simulink model "crazyflie_241010"  (R2024b)
settings: Solver=VariableStepAuto  StartTime=0.0  StopTime=10.0  RelTol=1e-3
model workspace (MAT data in the model file):
  CONFIG_CONTROLLER_PID_FILTER_ALL = Simulink.Parameter
  CONFIG_CONTROLLER_PID_FILTER_ALL.Complexity = 'real'
  CONFIG_CONTROLLER_PID_FILTER_ALL.Dimensions = [0 0]
  CONFIG_CONTROLLER_PID_FILTER_ALL.DataType = 'auto'
  a1 = Simulink.Parameter
  a1.Value = 2
  a1.Complexity = 'real'
  a1.Dimensions = [1 1]
  a1.DataType = 'auto'
  a2 = Simulink.Parameter
  a2.Value = 3
  a2.Complexity = 'real'
  a2.Dimensions = [1 1]
  a2.DataType = 'auto'
  b0 = Simulink.Parameter
  b0.Value = 5
  b0.Complexity = 'real'
  b0.Dimensions = [1 1]
  b0.DataType = 'auto'
  b1 = Simulink.Parameter
  b1.Value = 7
  b1.Complexity = 'real'
  b1.Dimensions = [1 1]
  b1.DataType = 'auto'
  b2 = Simulink.Parameter
  b2.Value = 11
  b2.Complexity = 'real'
  b2.Dimensions = [1 1]
  b2.DataType = 'auto'
  pid_dt = Simulink.Parameter
  pid_dt.Complexity = 'real'
  pid_dt.Dimensions = [0 0]
  pid_dt.DataType = 'auto'
  pid_enableDFilter = Simulink.Parameter
  pid_enableDFilter.Complexity = 'real'
  pid_enableDFilter.Dimensions = [0 0]
  pid_enableDFilter.DataType = 'auto'
  pid_iLimit = Simulink.Parameter
  pid_iLimit.Complexity = 'real'
  pid_iLimit.Dimensions = [0 0]
  pid_iLimit.DataType = 'auto'
  pid_kd = Simulink.Parameter
  pid_kd.Complexity = 'real'
  pid_kd.Dimensions = [0 0]
  pid_kd.DataType = 'auto'
  pid_kff = Simulink.Parameter
  pid_kff.Complexity = 'real'
  pid_kff.Dimensions = [0 0]
  pid_kff.DataType = 'auto'
  pid_ki = Simulink.Parameter
  pid_ki.Complexity = 'real'
  pid_ki.Dimensions = [0 0]
  pid_ki.DataType = 'auto'
  pid_kp = Simulink.Parameter
  pid_kp.Complexity = 'real'
  pid_kp.Dimensions = [0 0]
  pid_kp.DataType = 'auto'
  pid_outputLimit = Simulink.Parameter
  pid_outputLimit.Complexity = 'real'
  pid_outputLimit.Dimensions = [0 0]
  pid_outputLimit.DataType = 'auto'
settings Model: Creator=thomas  LastModifiedBy=thomas

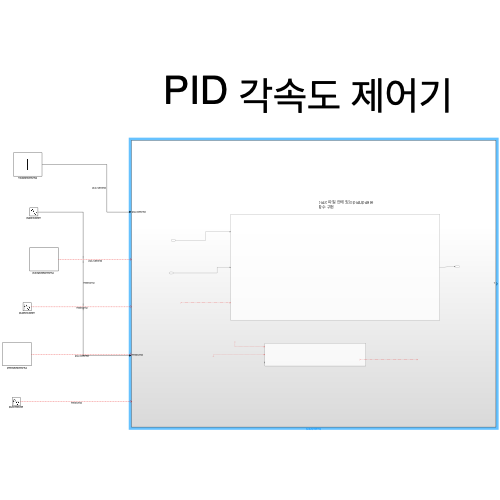
[thumbnail: Simulink's stored preview of the top-level diagram]
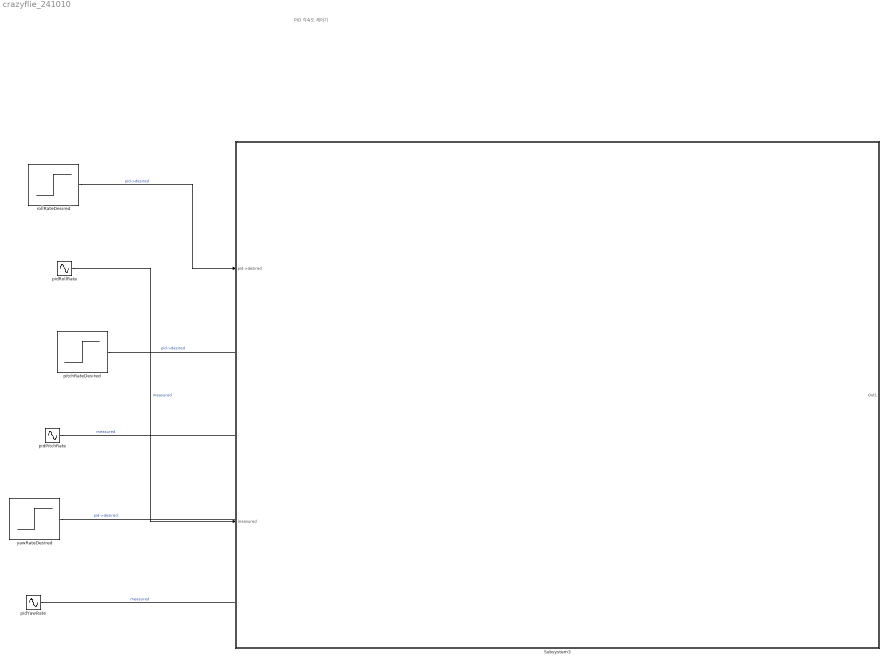
== system crazyflie_241010 ==
  note: PID 각속도 제어기
  Subsystem3 : Subsystem
  pidPitchRate : Sin  SampleTime=0
  pidRollRate : Sin  SampleTime=0
  pidYawRate : Sin  SampleTime=0
  "pitchRateDesired  " : Step  SampleTime=0
  rollRateDesired : Step  SampleTime=0
  yawRateDesired : Step  SampleTime=0
  wires:
  rollRateDesired/1 -> Subsystem3/1(pid->desired)  "pid->desired"
  pidRollRate/1 -> Subsystem3/2(measured)  "measured"
  "pitchRateDesired  "/1 -> ?  "pid->desired"
  pidPitchRate/1 -> ?  "measured"
  yawRateDesired/1 -> ?  "pid->desired"
  pidYawRate/1 -> ?  "measured"

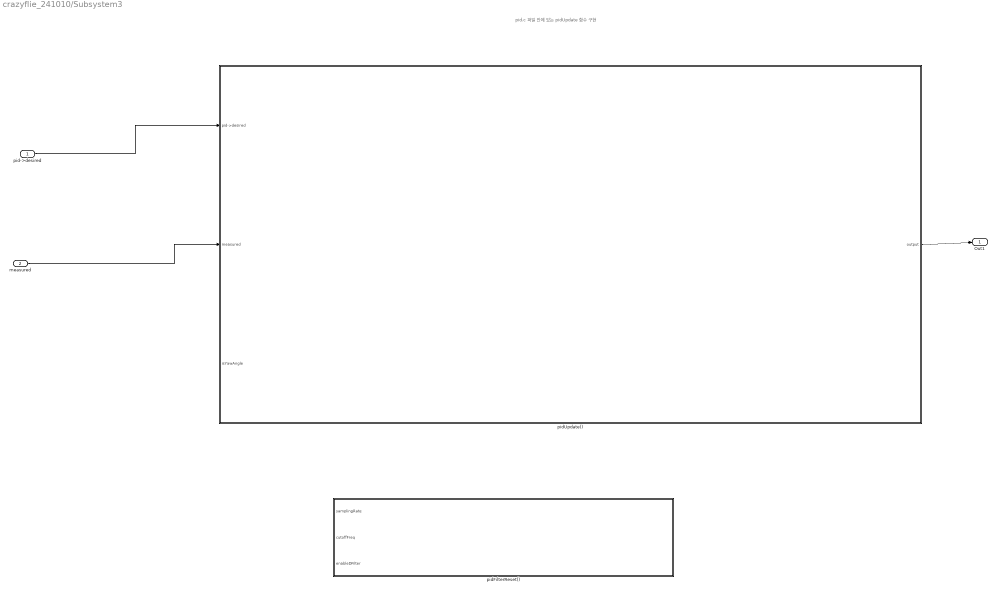
== system crazyflie_241010/Subsystem3 ==
  note: pid.c 파일 안에 있는 pidUpdate 함수 구현
  pid->desired : Inport
  measured : Inport  Port=2
  pidFilterReset() : Subsystem
  pidUpdate() : Subsystem
  Out1 : Outport
  wires:
  measured/1 -> pidUpdate()/2(measured)
  pid->desired/1 -> pidUpdate()/1(pid->desired)
  pidUpdate()/1(output) -> Out1/1
  ? -> pidUpdate()/3(isYawAngle)
  ? -> pidFilterReset()/1(samplingRate)
  ? -> ?
  ? -> pidFilterReset()/2(cutoffFreq)

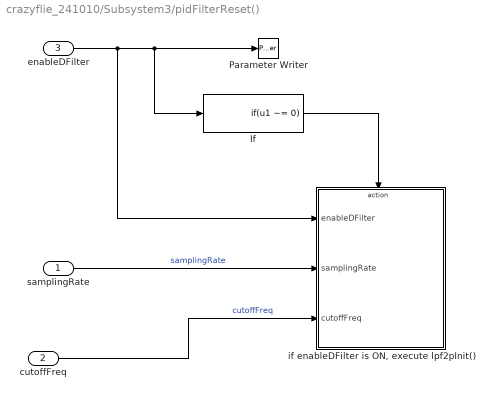
== system crazyflie_241010/Subsystem3/pidFilterReset() ==
  samplingRate : Inport
  cutoffFreq : Inport  Port=2
  enableDFilter : Inport  Port=3
  If : If  IfExpression=u1 ~= 0  ShowElse=off
  Parameter Writer : ParameterWriter  WorkspaceVariableName=pid_enableDFilter  Destination=Model workspace variable
  "if enableDFilter is ON, execute lpf2pInit()" : Subsystem  TreatAsAtomicUnit=on
  wires:
  samplingRate/1 -> "if enableDFilter is ON, execute lpf2pInit()"/2(samplingRate)  "samplingRate"
  enableDFilter/1 -> "if enableDFilter is ON, execute lpf2pInit()"/1(enableDFilter), If/1, Parameter Writer/1
  cutoffFreq/1 -> "if enableDFilter is ON, execute lpf2pInit()"/3(cutoffFreq)  "cutoffFreq"
  If/1 -> "if enableDFilter is ON, execute lpf2pInit()"/Action

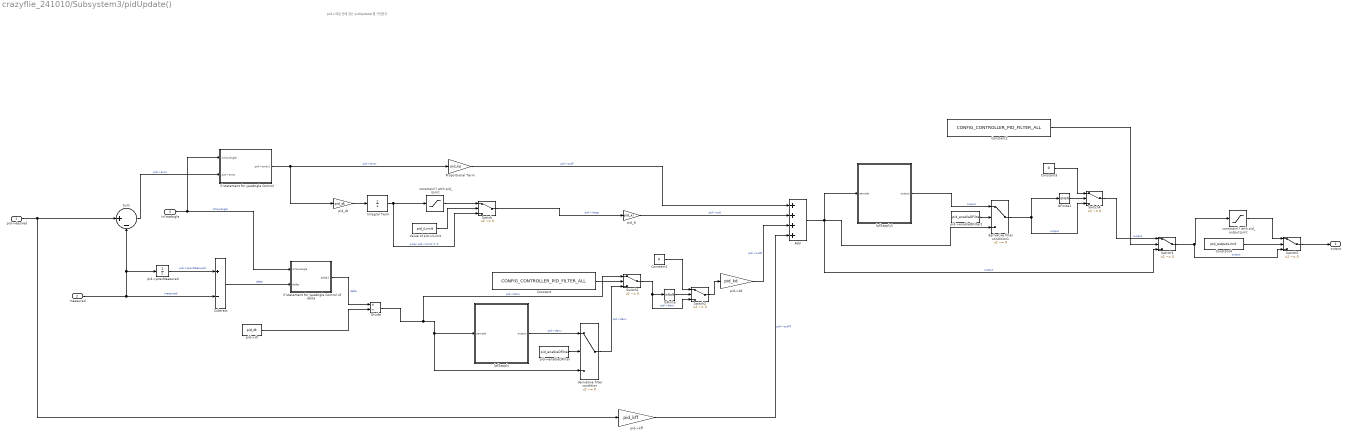
== system crazyflie_241010/Subsystem3/pidUpdate() ==
  note: pid.c 파일 안에 있는 pidUpdate()를 구현한것 .
  pid->desired : Inport
  measured : Inport  Port=2
  isYawAngle : Inport  Port=3
  Add : Sum  Inputs=++++
  Constant : Constant  Value=CONFIG_CONTROLLER_PID_FILTER_ALL
  Constant1 : Constant  Value=0
  Constant2 : Constant  Value=CONFIG_CONTROLLER_PID_FILTER_ALL
  Constant3 : Constant  Value=0
  Constant4 : Constant  Value=pid_outputLimit
  Divide : Product  Inputs=*/
  Integral Term : Integrator
  IsFinite : RelationalOperator  Operator=isNaN  OutDataTypeStr=boolean  RndMeth=Simplest  InputSameDT=off
  IsFinite1 : RelationalOperator  Operator=isNaN  OutDataTypeStr=boolean  RndMeth=Simplest  InputSameDT=off
  Proportional Term : Gain  Gain=pid_kp
  Subtract : Sum  Inputs=+-
  Sum : Sum  Inputs=|+-
  Switch{,1..5} (6 alike) : Switch  Criteria=u2 ~= 0  SaturateOnIntegerOverflow=off  InputSameDT=off
  Value of pid->iLimit : Constant  Value=pid_iLimit
  constrain() with pid_iLimit : Saturate  UpperLimit=pid_iLimit  LowerLimit=-pid_iLimit
  constrain() with pid_outputLimit : Saturate  UpperLimit=pid_outputLimit  LowerLimit=-pid_outputLimit
  derivative filter condition : Switch  Criteria=u2 ~= 0  Threshold=0.5  SaturateOnIntegerOverflow=off  InputSameDT=off
  derivative filter condition1 : Switch  Criteria=u2 ~= 0  Threshold=0.5  SaturateOnIntegerOverflow=off  InputSameDT=off
  "if statement for yawAngle Control " : Subsystem
  if statement for yawAngle Control of delta : Subsystem
  lpf2apply : Subsystem
  lpf2apply1 : Subsystem
  pid->dt : Constant  Value=pid_dt
  pid->enableDFilter : Constant  Value=pid_enableDFilter  LockScale=on
  pid->enableDFilter1 : Constant  Value=pid_enableDFilter  LockScale=on
  pid->kd : Gain  Gain=pid_kd
  pid->kff : Gain  Gain=pid_kff
  pid->prevMeasured : UnitDelay  SampleTime=-1  HasFrameUpgradeWarning=on
  pid_dt : Gain  Gain=pid_dt
  pid_ki : Gain  Gain=pid_ki
  output : Outport
  wires:
  pid->desired/1 -> pid->kff/1, Sum/1
  constrain() with pid_iLimit/1 -> Switch/1
  Integral Term/1 -> constrain() with pid_iLimit/1, Switch/3  "when pid->iLimit = 0"
  pid_dt/1 -> Integral Term/1
  pid->dt/1 -> Divide/2
  pid->kd/1 -> Add/3  "pid->outD"
  derivative filter condition/1 -> Switch1/3  "pid->deriv"
  Proportional Term/1 -> Add/1  "pid->outP"
  pid->prevMeasured/1 -> Subtract/1  "pid->prevMeasured"
  Value of pid->iLimit/1 -> Switch/2
  lpf2apply/1(output) -> derivative filter condition/1  "pid->deriv"
  Switch/1 -> pid_ki/1  "pid->integ"
  Subtract/1 -> if statement for yawAngle Control of delta/2(delta)  "delta"
  measured/1 -> Sum/2, pid->prevMeasured/1, Subtract/2  "measured"
  pid_ki/1 -> Add/2  "pid->outI"
  pid->enableDFilter/1 -> derivative filter condition/2
  "if statement for yawAngle Control "/1(pid->error1) -> Proportional Term/1, pid_dt/1  "pid->error"
  isYawAngle/1 -> "if statement for yawAngle Control "/1(isYawAngle), if statement for yawAngle Control of delta/1(isYawAngle)  "isYawAngle"
  Sum/1 -> "if statement for yawAngle Control "/2(pid->error)  "pid->error"
  if statement for yawAngle Control of delta/1(delta1) -> Divide/1  "delta"
  pid->kff/1 -> Add/4  "pid->outFF"
  Constant/1 -> Switch1/2
  Divide/1 -> derivative filter condition/3, lpf2apply/1(sample), Switch1/1  "pid->deriv"
  Switch1/1 -> Switch2/3, IsFinite/1  "pid->deriv"
  IsFinite/1 -> Switch2/2
  Constant1/1 -> Switch2/1
  Switch2/1 -> pid->kd/1
  Add/1 -> lpf2apply1/1(sample), derivative filter condition1/3, Switch3/3  "output"
  pid->enableDFilter1/1 -> derivative filter condition1/2
  Constant3/1 -> Switch4/1
  IsFinite1/1 -> Switch4/2
  lpf2apply1/1(output) -> derivative filter condition1/1  "output"
  derivative filter condition1/1 -> Switch4/3, IsFinite1/1  "output"
  Constant2/1 -> Switch3/2
  Switch4/1 -> Switch3/1  "output"
  Constant4/1 -> Switch5/2
  Switch3/1 -> Switch5/3, constrain() with pid_outputLimit/1  "output"
  constrain() with pid_outputLimit/1 -> Switch5/1
  Switch5/1 -> output/1

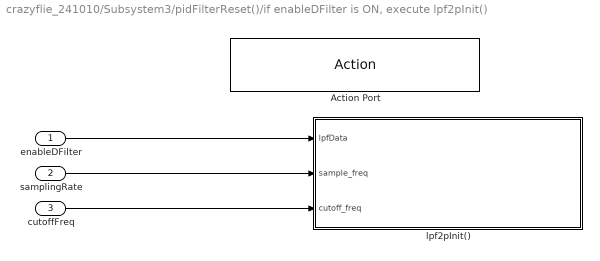
== system crazyflie_241010/Subsystem3/pidFilterReset()/if enableDFilter is ON, execute lpf2pInit() ==
  enableDFilter : Inport
  samplingRate : Inport  Port=2
  cutoffFreq : Inport  Port=3
  Action Port : ActionPort  ActionPortLabel=if(u1 ~= 0)
  lpf2pInit() : Subsystem
  wires:
  enableDFilter/1 -> lpf2pInit()/1(lpfData)
  samplingRate/1 -> lpf2pInit()/2(sample_freq)
  cutoffFreq/1 -> lpf2pInit()/3(cutoff_freq)

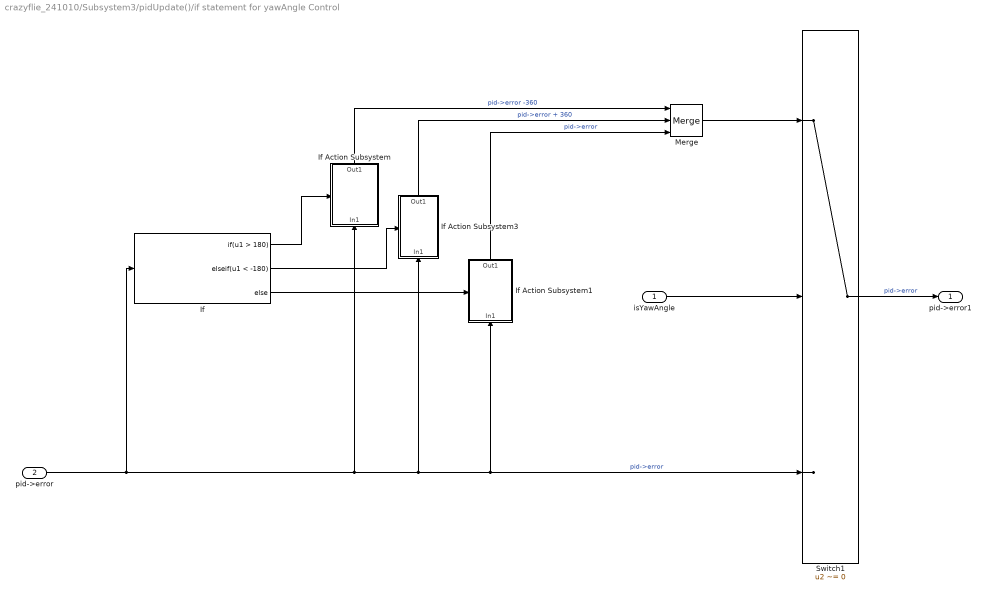
== system crazyflie_241010/Subsystem3/pidUpdate()/if statement for yawAngle Control  ==
  isYawAngle : Inport
  pid->error : Inport  Port=2
  If : If  IfExpression=u1 > 180  ElseIfExpressions=u1 < -180
  If Action Subsystem : Subsystem  TreatAsAtomicUnit=on
  If Action Subsystem1 : Subsystem  TreatAsAtomicUnit=on
  If Action Subsystem3 : Subsystem  TreatAsAtomicUnit=on
  Merge : Merge  Inputs=3
  Switch1 : Switch  Criteria=u2 ~= 0  Threshold=0.5  SaturateOnIntegerOverflow=off  InputSameDT=off
  pid->error1 : Outport
  wires:
  If Action Subsystem3/1(Out1) -> Merge/2  "pid->error + 360"
  Merge/1 -> Switch1/1
  Switch1/1 -> pid->error1/1  "pid->error"
  isYawAngle/1 -> Switch1/2
  pid->error/1 -> If Action Subsystem1/1(In1), Switch1/3, If Action Subsystem3/1(In1), If Action Subsystem/1(In1), If/1  "pid->error"
  If/3 -> If Action Subsystem1/Action
  If Action Subsystem1/1(Out1) -> Merge/3  "pid->error"
  If/1 -> If Action Subsystem/Action
  If Action Subsystem/1(Out1) -> Merge/1  "pid->error -360"
  If/2 -> If Action Subsystem3/Action

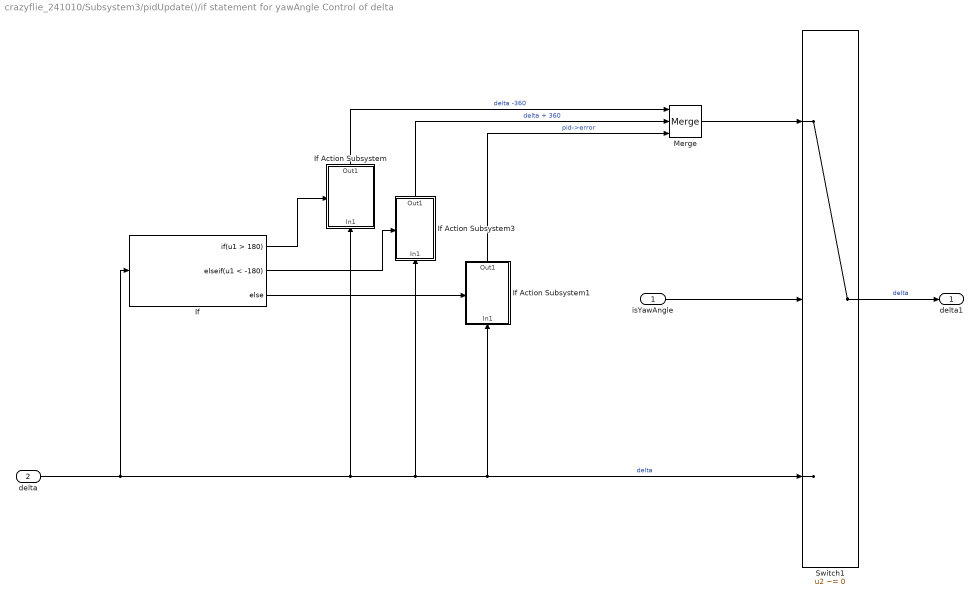
== system crazyflie_241010/Subsystem3/pidUpdate()/if statement for yawAngle Control of delta ==
  isYawAngle : Inport
  delta : Inport  Port=2
  If : If  IfExpression=u1 > 180  ElseIfExpressions=u1 < -180
  If Action Subsystem : Subsystem  TreatAsAtomicUnit=on
  If Action Subsystem1 : Subsystem  TreatAsAtomicUnit=on
  If Action Subsystem3 : Subsystem  TreatAsAtomicUnit=on
  Merge : Merge  Inputs=3
  Switch1 : Switch  Criteria=u2 ~= 0  Threshold=0.5  SaturateOnIntegerOverflow=off  InputSameDT=off
  delta1 : Outport
  wires:
  If Action Subsystem3/1(Out1) -> Merge/2  "delta + 360"
  Merge/1 -> Switch1/1
  Switch1/1 -> delta1/1  "delta"
  isYawAngle/1 -> Switch1/2
  delta/1 -> If Action Subsystem1/1(In1), Switch1/3, If Action Subsystem3/1(In1), If Action Subsystem/1(In1), If/1  "delta"
  If/3 -> If Action Subsystem1/Action
  If Action Subsystem1/1(Out1) -> Merge/3  "pid->error"
  If/1 -> If Action Subsystem/Action
  If Action Subsystem/1(Out1) -> Merge/1  "delta -360"
  If/2 -> If Action Subsystem3/Action

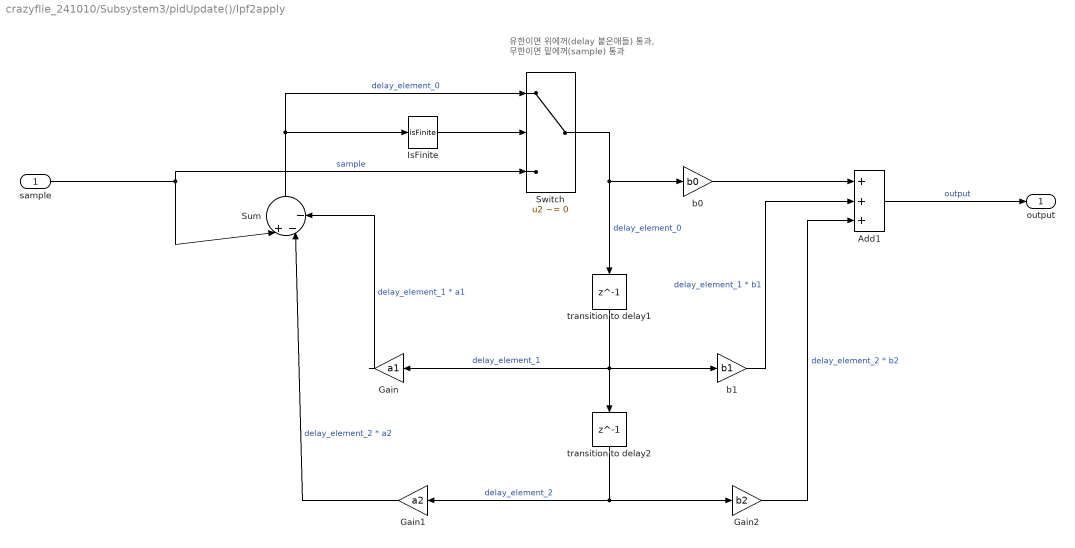
== system crazyflie_241010/Subsystem3/pidUpdate()/lpf2apply ==
  note: 유한이면 위에꺼(delay 붙은애들) 통과,
      | 무한이면 밑에꺼(sample) 통과
  sample : Inport
  Add1 : Sum  Inputs=+++
  Gain : Gain  Gain=a1
  Gain1 : Gain  Gain=a2
  Gain2 : Gain  Gain=b2
  IsFinite : RelationalOperator  Operator=isFinite  OutDataTypeStr=boolean  RndMeth=Simplest  InputSameDT=off
  Sum : Sum  Inputs=|+--
  Switch : Switch  Criteria=u2 ~= 0  Threshold=99999999  SaturateOnIntegerOverflow=off  InputSameDT=off
  b0 : Gain  Gain=b0
  b1 : Gain  Gain=b1
  transition to delay1 : Delay  DelayLength=1  InitialCondition=0
  transition to delay2 : Delay  DelayLength=1  InitialCondition=0
  output : Outport
  wires:
  transition to delay2/1 -> Gain1/1, Gain2/1  "delay_element_2"
  b1/1 -> Add1/2  "delay_element_1 * b1"
  Gain1/1 -> Sum/2  "delay_element_2 * a2"
  Gain/1 -> Sum/3  "delay_element_1 * a1"
  IsFinite/1 -> Switch/2
  sample/1 -> Sum/1, Switch/3  "sample"
  Sum/1 -> Switch/1, IsFinite/1  "delay_element_0"
  Gain2/1 -> Add1/3  "delay_element_2 * b2"
  Add1/1 -> output/1  "output"
  Switch/1 -> transition to delay1/1, b0/1  "delay_element_0"
  b0/1 -> Add1/1
  transition to delay1/1 -> Gain/1, b1/1, transition to delay2/1  "delay_element_1"

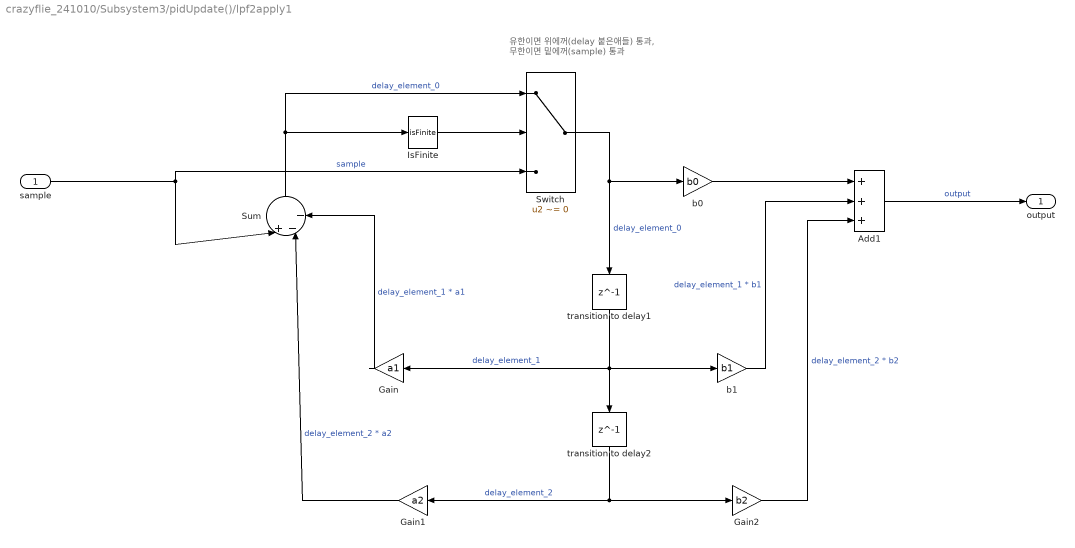
== system crazyflie_241010/Subsystem3/pidUpdate()/lpf2apply1 ==
  note: 유한이면 위에꺼(delay 붙은애들) 통과,
      | 무한이면 밑에꺼(sample) 통과
  sample : Inport
  Add1 : Sum  Inputs=+++
  Gain : Gain  Gain=a1
  Gain1 : Gain  Gain=a2
  Gain2 : Gain  Gain=b2
  IsFinite : RelationalOperator  Operator=isFinite  OutDataTypeStr=boolean  RndMeth=Simplest  InputSameDT=off
  Sum : Sum  Inputs=|+--
  Switch : Switch  Criteria=u2 ~= 0  Threshold=99999999  SaturateOnIntegerOverflow=off  InputSameDT=off
  b0 : Gain  Gain=b0
  b1 : Gain  Gain=b1
  transition to delay1 : Delay  DelayLength=1  InitialCondition=0
  transition to delay2 : Delay  DelayLength=1  InitialCondition=0
  output : Outport
  wires:
  transition to delay2/1 -> Gain1/1, Gain2/1  "delay_element_2"
  b1/1 -> Add1/2  "delay_element_1 * b1"
  Gain1/1 -> Sum/2  "delay_element_2 * a2"
  Gain/1 -> Sum/3  "delay_element_1 * a1"
  IsFinite/1 -> Switch/2
  sample/1 -> Sum/1, Switch/3  "sample"
  Sum/1 -> Switch/1, IsFinite/1  "delay_element_0"
  Gain2/1 -> Add1/3  "delay_element_2 * b2"
  Add1/1 -> output/1  "output"
  Switch/1 -> transition to delay1/1, b0/1  "delay_element_0"
  b0/1 -> Add1/1
  transition to delay1/1 -> Gain/1, b1/1, transition to delay2/1  "delay_element_1"

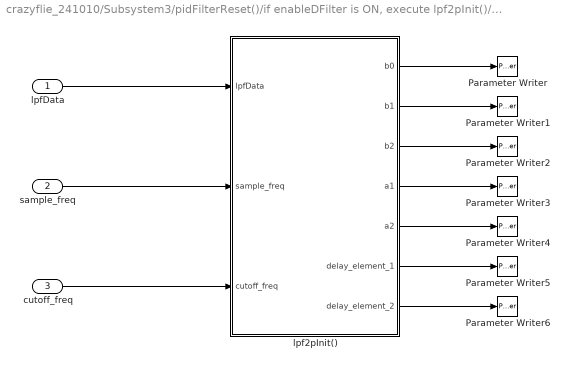
== system crazyflie_241010/Subsystem3/pidFilterReset()/if enableDFilter is ON, execute lpf2pInit()/lpf2pInit() ==
  lpfData : Inport
  sample_freq : Inport  Port=2
  cutoff_freq : Inport  Port=3
  Parameter Writer : ParameterWriter  WorkspaceVariableName=b0  Destination=Model workspace variable
  Parameter Writer1 : ParameterWriter  WorkspaceVariableName=b1  Destination=Model workspace variable
  Parameter Writer2 : ParameterWriter  WorkspaceVariableName=b2  Destination=Model workspace variable
  Parameter Writer3 : ParameterWriter  WorkspaceVariableName=a1  Destination=Model workspace variable
  Parameter Writer4 : ParameterWriter  WorkspaceVariableName=a2  Destination=Model workspace variable
  Parameter Writer5 : ParameterWriter  WorkspaceVariableName=delay_element_1  Destination=Model workspace variable
  Parameter Writer6 : ParameterWriter  WorkspaceVariableName=delay_element_2  Destination=Model workspace variable
  lpf2pInit() : MATLAB Function  TreatAsAtomicUnit=on
  wires:
  lpfData/1 -> lpf2pInit()/1(lpfData)
  lpf2pInit()/1(b0) -> Parameter Writer/1
  lpf2pInit()/2(b1) -> Parameter Writer1/1
  lpf2pInit()/3(b2) -> Parameter Writer2/1
  lpf2pInit()/4(a1) -> Parameter Writer3/1
  lpf2pInit()/5(a2) -> Parameter Writer4/1
  lpf2pInit()/6(delay_element_1) -> Parameter Writer5/1
  lpf2pInit()/7(delay_element_2) -> Parameter Writer6/1
  sample_freq/1 -> lpf2pInit()/2(sample_freq)
  cutoff_freq/1 -> lpf2pInit()/3(cutoff_freq)

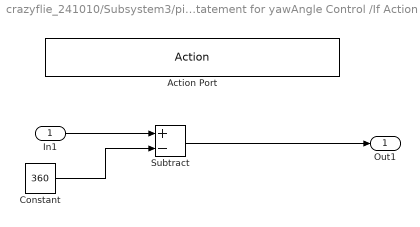
== system crazyflie_241010/Subsystem3/pidUpdate()/if statement for yawAngle Control /If Action Subsystem ==
  In1 : Inport
  Action Port : ActionPort  ActionPortLabel=if(u1 > 180)
  Constant : Constant  Value=360
  Subtract : Sum  Inputs=+-
  Out1 : Outport
  wires:
  In1/1 -> Subtract/1
  Constant/1 -> Subtract/2
  Subtract/1 -> Out1/1

== system crazyflie_241010/Subsystem3/pidUpdate()/if statement for yawAngle Control /If Action Subsystem1 ==
  In1 : Inport
  Action Port : ActionPort  ActionPortLabel=else
  Out1 : Outport
  wires:
  In1/1 -> Out1/1

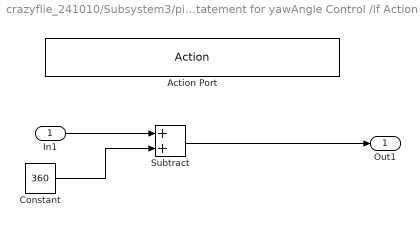
== system crazyflie_241010/Subsystem3/pidUpdate()/if statement for yawAngle Control /If Action Subsystem3 ==
  In1 : Inport
  Action Port : ActionPort  ActionPortLabel=elseif(u1 < -180)
  Constant : Constant  Value=360
  Subtract : Sum
  Out1 : Outport
  wires:
  In1/1 -> Subtract/1
  Constant/1 -> Subtract/2
  Subtract/1 -> Out1/1

== system crazyflie_241010/Subsystem3/pidUpdate()/if statement for yawAngle Control of delta/If Action Subsystem ==
  In1 : Inport
  Action Port : ActionPort
  Constant : Constant  Value=360
  Subtract : Sum  Inputs=+-
  Out1 : Outport
  wires:
  In1/1 -> Subtract/1
  Constant/1 -> Subtract/2
  Subtract/1 -> Out1/1

== system crazyflie_241010/Subsystem3/pidUpdate()/if statement for yawAngle Control of delta/If Action Subsystem1 ==
  In1 : Inport
  Action Port : ActionPort
  Out1 : Outport
  wires:
  In1/1 -> Out1/1

== system crazyflie_241010/Subsystem3/pidUpdate()/if statement for yawAngle Control of delta/If Action Subsystem3 ==
  In1 : Inport
  Action Port : ActionPort
  Constant : Constant  Value=360
  Subtract : Sum
  Out1 : Outport
  wires:
  In1/1 -> Subtract/1
  Constant/1 -> Subtract/2
  Subtract/1 -> Out1/1

== matlab function crazyflie_241010/Subsystem3/pidFilterReset()/if enableDFilter is ON, execute lpf2pInit()/lpf2pInit()/lpf2pInit() ==
  data: lpfData input; b0 output; sample_freq input; cutoff_freq input; b1 output; b2 output; a1 output; a2 output; delay_element_1 output; delay_element_2 output
function [b0,b1,b2,a1,a2,delay_element_1,delay_element_2] = lpf2pInit(lpfData, sample_freq,cutoff_freq)

if cutoff_freq <= 0 
    return;
end

if sample_freq <= 0
    return;
end

[b0,b1,b2,a1,a2,delay_element_1,delay_element_2]=lpf2pSetCutoffFreq(lpfData, sample_freq, cutoff_freq)
